simulink model "Untitled2"  (R2013b)
settings: Solver=ode4  StartTime=0.0  StopTime=tSim  FixedStep=h  RelTol=1e-3
values from neighbouring files (symbols this model uses):
  y0 = 0    [launcher.m]    (also in launcher2.m = 1)
settings Model: Creator=JAR  LastModifiedBy=JAR

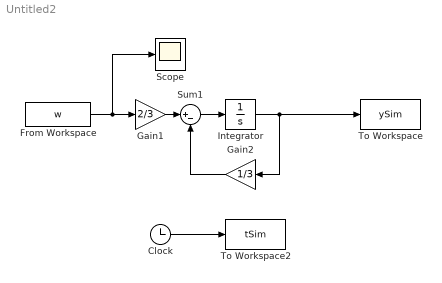
== system Untitled2 ==
  Clock : Clock
  From Workspace : FromWorkspace  VariableName=w  SampleTime=0
  Gain1 : Gain  Gain=2/3
  Gain2 : Gain  Gain=1/3
  Integrator : Integrator  InitialCondition=y0
  Scope : Scope
  Sum1 : Sum  Inputs=|+-
  To Workspace : ToWorkspace  VariableName=ySim  SampleTime=-1
  To Workspace2 : ToWorkspace  VariableName=tSim  SampleTime=-1
  wires:
  Clock/1 -> To Workspace2/1
  Gain1/1 -> Sum1/1
  Gain2/1 -> Sum1/2
  Sum1/1 -> Integrator/1
  Integrator/1 -> To Workspace/1, Gain2/1
  From Workspace/1 -> Scope/1, Gain1/1
